simulink model "powerwindow_tl"  (R2021a)
settings: Solver=ode3  StartTime=0.0  StopTime=inf  FixedStep=0.01  RelTol=1e-3  EnableMultiTasking=on
PreLoadFcn:
  | if exist('tl_preloadfcn','file'), tl_preloadfcn(gcs,'5.2.0.25'); end
PostLoadFcn:
  | , if any(exist('dsrtsu_mdlpostloadfcn', 'file') == [2, 3, 6]), try dsrtsu_mdlpostloadfcn('Execute', bdroot); catch fprintf('Error in PostLoadFcn (dsrtsu_mdlpostloadfcn) for model "%s":\n %s\n', bdroot, lasterr); end, end,
  | if exist('tl_postloadfcn','file'), tl_postloadfcn(gcs,'5.2.0.25'); end
InitFcn:
  | , if any(exist('rtifpga_mdlclblib', 'file') ~= 0), rtifpga_mdlclblib('Init', bdroot); end,
  | if exist('tlds_init','file'), tlds_init(gcs); end
StartFcn:
  | if exist('tlds_start','file'), tlds_start(gcs); end
StopFcn:
  | if exist('tlds_stop','file'), tlds_stop(gcs); end
model workspace (MAT data in the model file):
  obs_1 = 1
  obs_10 = 1
  obs_11 = 1
  obs_12 = 1
  obs_13 = 1
  obs_14 = 1
  obs_15 = 1
  obs_16 = 1
  obs_17 = 1
  obs_18 = 1
  obs_19 = 1
  obs_2 = 1
  obs_20 = 1
  obs_21 = 1
  obs_22 = 1
  obs_23 = 1
  obs_24 = 1
  obs_25 = 1
  obs_26 = 1
  obs_27 = 1
  obs_28 = 1
  obs_29 = 1
  obs_3 = 1
  obs_30 = 1
  obs_31 = 1
  obs_32 = 1
  obs_4 = 1
  obs_5 = 1
  obs_6 = 1
  obs_7 = 1
  obs_8 = 1
  obs_9 = 1
values from neighbouring files (symbols this model uses):
  auto_down_time = 100    [powerwindow_tl_init.m]    (also in test_init.m = copy(auto_up_time))
  auto_up_time = 100    [powerwindow_tl_init.m]    (also in test_init.m = Simulink.Parameter)
  emergency_down_time = 100    [powerwindow_tl_init.m]    (also in test_init.m = copy(auto_up_time))
  position_endstop_top = 0.4    [powerwindow_tl_init.m]    (also in test_init.m = Simulink.Parameter)
undefined symbols (not defined in the file or in its folder): DiscIntNeverNeededParam
libraries: tllib x3, powerwindow_blocklib x2
PreSaveFcn:
  | if exist('tl_presavefcn','file'), tl_presavefcn(gcs); end
CloseFcn:
  | if exist('tl_closefcn','file'), tl_closefcn(gcs); end
settings Model: DSRTSU_INTERNAL_RTI_VER=590  DSRTSU_INTERNAL_RTI_TYPE=rti1006  DSRTSU_INTERNAL_RTIFPGA=170  RTICANMMDATA=struct('GeneralSetupData',struct('modelroot','C:\PowerWindowDemo_TL52_22.0J','generalsettings',struct('filesettings',struct('destfolder',struct('Name','RTICANMM_FILES','Check',1),'buildfolder',struct('Name','.','Check',1),'AbsDestfolder',struct('Name','C:\PowerWindowDemo_TL52_22.0J\RTICANMM_FILES'),'AbsBuildfolder',struct('Name','C:\PowerWindowDemo_TL52_22.0J'))),'options',struct('addpaths',1,'rmpaths',1,'addtrcexclusion',true,'cannavigator',struct('checkmonitoring',0),'show_usrtrc',0,'use_usrtrc',0),'advanced',struct('options',ones(1,100)),'MPSetup',{{}},'RTI',struct('Type','ERT','Ver','','Date',''),'modelname','powerwindow_tl','block','powerwindow_tl'))  TL_MAIN_DATA={'date',738790.66649789352}  DS_PROJECTFILE=sample.dd  TLVersion=5.2.0.25  DSRTSU_INTERNAL_RTISTBM_VER=1.4.3  Creator=hholberg  LastModifiedBy=BTCJ_support
settings SolverCC: AlgebraicLoopSolver=TrustRegion
settings DataIOCC: LimitDataPoints=on  SaveFormat=StructureWithTime  ReturnWorkspaceOutputs=off
settings OptimizationCC: BlockReduction=off  OptimizeBlockIOStorage=off  BufferReuse=off  GlobalBufferReuse=off  ExpressionFolding=off  EnableMemcpy=off  ExpressionDepthLimit=2147483647  LocalBlockOutputs=off  ZeroExternalMemoryAtStartup=off  ZeroInternalMemoryAtStartup=off  InitFltsAndDblsToZero=on  LifeSpan=Inf  OptimizeDataStoreBuffers=off  BusAssignmentInplaceUpdate=off  EfficientTunableParamExpr=on
settings DebuggingCC: UnderspecifiedInitializationDetection=Classic  MergeDetectMultiDrivingBlocksExec=none  SolverPrmCheckMsg=warning  FcnCallInpInsideContextMsg=warning  BusObjectLabelMismatch=error  StateNameClashWarn=warning  StrictBusMsg=ErrorOnBusTreatedAsVector  NonBusSignalsTreatedAsBus=error  SFUnexpectedBacktrackingDiag=warning  SFNoUnconditionalDefaultTransitionDiag=warning  SFExecutionAtInitializationDiag=none  SFMachineParentedDataDiag=warning  ArithmeticOperatorsInVariantConditions=warning
settings HardwareCC: ProdBitPerPointer=32  ProdBitPerSizeT=32  ProdBitPerPtrDiffT=32  ProdLargestAtomicInteger=Integer  ProdEndianess=Unspecified  ProdWordSize=32  ProdHWDeviceType=32-bit Generic  TargetIntDivRoundTo=Zero  TargetEndianess=LittleEndian  TargetHWDeviceType=Custom Processor->Custom
settings ModelReferenceCC: PropagateSignalLabelsOutOfModel=off
settings SFSimCC: SimUseLocalCustomCode=off  MATLABDynamicMemAlloc=off  CustomCodeUndefinedFunction=UseInterfaceOnly
settings RTWCC: SystemTargetFile=ert.tlc  GenCodeOnly=on  TemplateMakefile=ert_default_tmf  RTWUseLocalCustomCode=off
settings CodeAppCC: IgnoreCustomStorageClasses=off  StateflowObjectComments=on  InternalIdentifier=Classic
settings ERTTargetCC: MultiwordLength=2048  ERTCustomFileTemplate=example_file_process.tlc  ConvertIfToSwitch=off  SuppressUnreachableDefaultCases=off
settings ConfigComp: CovMetricSettings=dw  CovSaveCumulativeToWorkspaceVar=on  CovSaveSingleToWorkspaceVar=on  CovExternalEMLEnable=off

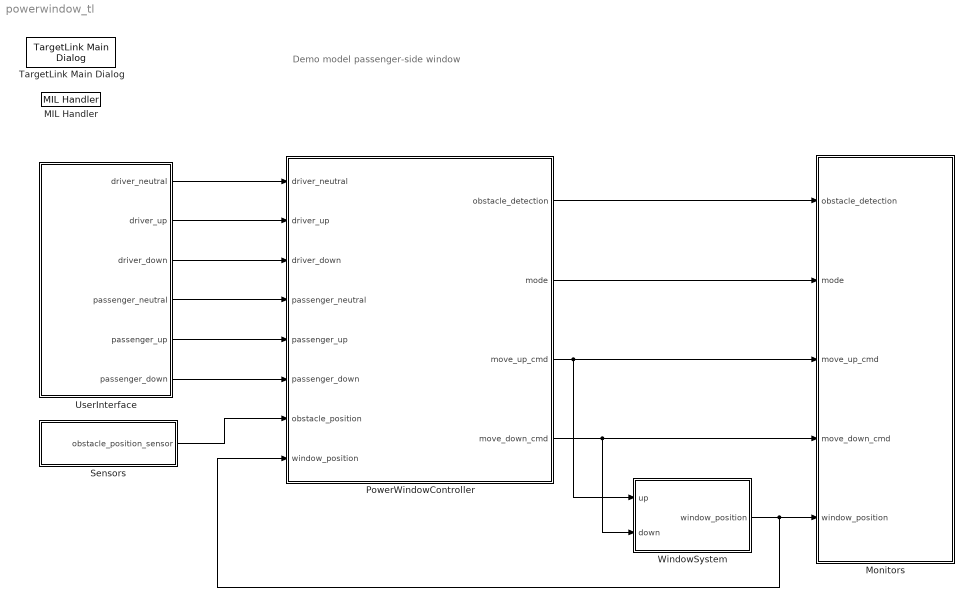
== system powerwindow_tl ==
  note: Demo model passenger-side window
  MIL Handler : tllib/MIL Handler  data={'date',730486}
      settings: SourceProductName=dSPACE TargetLink common blockset
  Monitors : Subsystem
  PowerWindowController : Subsystem  Tag=TargetLink Simulation Frame  mask(TL_SimFrame){}
      settings: CopyFcn=if exist('tl_copyfcn','file'), tl_copyfcn(gcbh); end  NameChangeFcn=if exist('tl_framenamechangefcn','file'), tl_framenamechangefcn(gcbh); end
      settings: OpenFcn=|
      | if exist('open_tlsubsystem','file')
      |    open_tlsubsystem(gcbh);
      | else
      |    tlsubsystem = ...
      |       find_system(gcb, ...
      |       'LookUnderMasks','on', ...
      |       'FollowLinks','on', ...
      |       'Tag','MIL Subsystem');
      |    open_system(tlsubsystem);
      | end
      mask Display: disp('TargetLink\nModel-\nin-the-loop\nmode')
  Sensors : Subsystem
  TargetLink Main Dialog : tllib/TargetLink Main Dialog  data=[]
      settings: SourceProductName=dSPACE TargetLink common blockset
  UserInterface : Subsystem
  WindowSystem : Subsystem
  wires:
  PowerWindowController/3(move_up_cmd) -> WindowSystem/1(up), Monitors/3(move_up_cmd)
  PowerWindowController/4(move_down_cmd) -> Monitors/4(move_down_cmd), WindowSystem/2(down)
  WindowSystem/1(window_position) -> PowerWindowController/8(window_position), Monitors/5(window_position)
  UserInterface/1(driver_neutral) -> PowerWindowController/1(driver_neutral)
  UserInterface/2(driver_up) -> PowerWindowController/2(driver_up)
  UserInterface/3(driver_down) -> PowerWindowController/3(driver_down)
  UserInterface/4(passenger_neutral) -> PowerWindowController/4(passenger_neutral)
  UserInterface/5(passenger_up) -> PowerWindowController/5(passenger_up)
  UserInterface/6(passenger_down) -> PowerWindowController/6(passenger_down)
  Sensors/1(obstacle_position_sensor) -> PowerWindowController/7(obstacle_position)
  PowerWindowController/1(obstacle_detection) -> Monitors/1(obstacle_detection)
  PowerWindowController/2(mode) -> Monitors/2(mode)

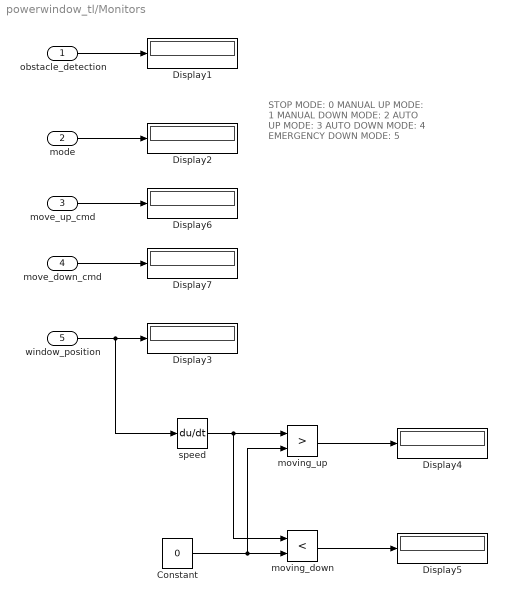
== system powerwindow_tl/Monitors ==
  note: STOP MODE: 0
      | MANUAL UP MODE: 1
      | MANUAL DOWN MODE: 2
      | AUTO UP MODE: 3
      | AUTO DOWN MODE: 4
      | EMERGENCY DOWN MODE: 5
  obstacle_detection : Inport
  mode : Inport  Port=2
  move_up_cmd : Inport  Port=3
  move_down_cmd : Inport  Port=4
  window_position : Inport  Port=5
  Constant : Constant  Value=0
  Display{1..7} (7 alike) : Display
  moving_down : RelationalOperator  Operator=<  OutDataTypeStr=boolean  RndMeth=Nearest
  moving_up : RelationalOperator  Operator=>  OutDataTypeStr=boolean  RndMeth=Nearest
  speed : Derivative
  wires:
  obstacle_detection/1 -> Display1/1
  mode/1 -> Display2/1
  window_position/1 -> speed/1, Display3/1
  speed/1 -> moving_down/1, moving_up/1
  Constant/1 -> moving_down/2, moving_up/2
  moving_down/1 -> Display5/1
  moving_up/1 -> Display4/1
  move_up_cmd/1 -> Display6/1
  move_down_cmd/1 -> Display7/1

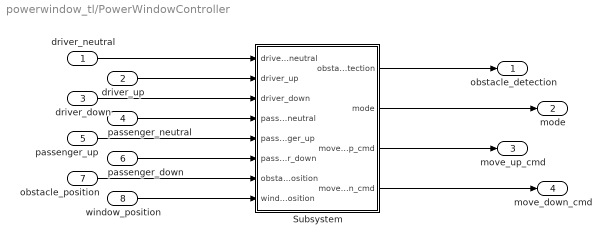
== system powerwindow_tl/PowerWindowController ==
  driver_neutral : Inport
  driver_up : Inport  Port=2
  driver_down : Inport  Port=3
  passenger_neutral : Inport  Port=4
  passenger_up : Inport  Port=5
  passenger_down : Inport  Port=6
  obstacle_position : Inport  Port=7
  window_position : Inport  Port=8
  Subsystem : Subsystem  Tag=struct('sfcnName','PowerWindowController_sf','subFunction','','srcSubsystem','')  mask(TL_Enable){}
      settings: OpenFcn=warndlg(get_param(gcb,'MaskHelp'),'Serious Warning');
      mask Help: This subsystem keeps the TargetLink subsystem (subsystem with TargetLink blocks for production code generation), and is needed for the TargetLink simulation frame to work properly. DO NOT DELETE OR MODIFY IT!
  obstacle_detection : Outport
  mode : Outport  Port=2  OutDataTypeStr=uint8
  move_up_cmd : Outport  Port=3
  move_down_cmd : Outport  Port=4
  wires:
  driver_neutral/1 -> Subsystem/1(driver_neutral)
  driver_up/1 -> Subsystem/2(driver_up)
  driver_down/1 -> Subsystem/3(driver_down)
  passenger_neutral/1 -> Subsystem/4(passenger_neutral)
  passenger_up/1 -> Subsystem/5(passenger_up)
  passenger_down/1 -> Subsystem/6(passenger_down)
  obstacle_position/1 -> Subsystem/7(obstacle_position)
  window_position/1 -> Subsystem/8(window_position)
  Subsystem/1(obstacle_detection) -> obstacle_detection/1
  Subsystem/2(mode) -> mode/1
  Subsystem/3(move_up_cmd) -> move_up_cmd/1
  Subsystem/4(move_down_cmd) -> move_down_cmd/1

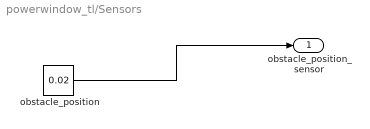
== system powerwindow_tl/Sensors ==
  obstacle_position : Constant  Value=0.02  OutDataTypeStr=double
  obstacle_position_sensor : Outport
  wires:
  obstacle_position/1 -> obstacle_position_sensor/1

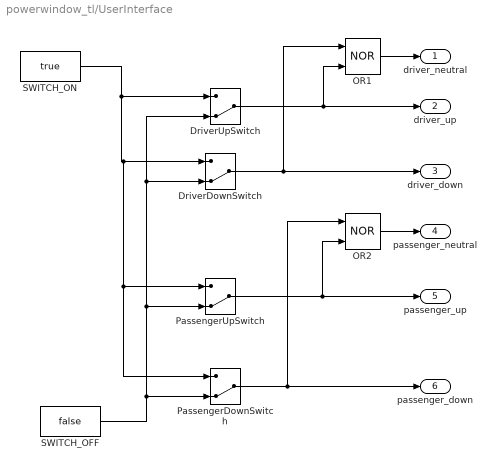
== system powerwindow_tl/UserInterface ==
  DriverDownSwitch : ManualSwitch  CurrentSetting=0
  DriverUpSwitch : ManualSwitch  CurrentSetting=0
  OR1 : Logic  Operator=NOR  AllPortsSameDT=off  OutDataTypeStr=boolean
  OR2 : Logic  Operator=NOR  AllPortsSameDT=off  OutDataTypeStr=boolean
  PassengerDownSwitch : ManualSwitch  CurrentSetting=0
  PassengerUpSwitch : ManualSwitch  CurrentSetting=0
  SWITCH_OFF : Constant  Value=false  OutDataTypeStr=boolean
  SWITCH_ON : Constant  Value=true  OutDataTypeStr=boolean
  driver_neutral : Outport
  driver_up : Outport  Port=2
  driver_down : Outport  Port=3
  passenger_neutral : Outport  Port=4
  passenger_up : Outport  Port=5
  passenger_down : Outport  Port=6
  wires:
  SWITCH_ON/1 -> PassengerDownSwitch/1, PassengerUpSwitch/1, DriverDownSwitch/1, DriverUpSwitch/1
  SWITCH_OFF/1 -> DriverUpSwitch/2, DriverDownSwitch/2, PassengerUpSwitch/2, PassengerDownSwitch/2
  DriverUpSwitch/1 -> OR1/2, driver_up/1
  DriverDownSwitch/1 -> OR1/1, driver_down/1
  OR1/1 -> driver_neutral/1
  PassengerUpSwitch/1 -> OR2/2, passenger_up/1
  PassengerDownSwitch/1 -> OR2/1, passenger_down/1
  OR2/1 -> passenger_neutral/1

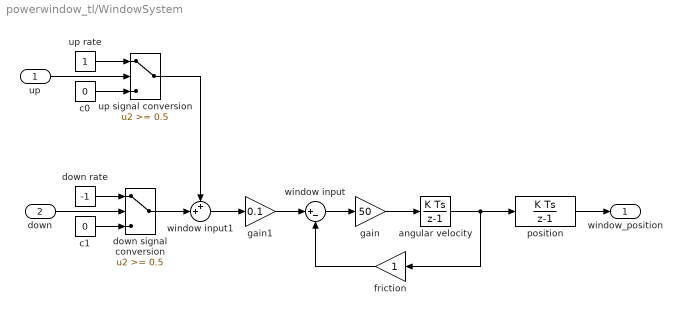
== system powerwindow_tl/WindowSystem ==
  up : Inport
  down : Inport  Port=2
  angular velocity : DiscreteIntegrator  SampleTime=0.01  ICPrevOutput=DiscIntNeverNeededParam  ICPrevScaledInput=DiscIntNeverNeededParam  mask(DiscretizedDiscreteIntegrator){}
      mask init:
      | %zoh
  c0 : Constant  Value=0
  c1 : Constant  Value=0
  down rate : Constant  Value=-1
  down signal conversion : Switch  Threshold=0.5  InputSameDT=on
  friction : Gain  SaturateOnIntegerOverflow=on  OutDataTypeStr=Inherit: Same as input  ParamDataTypeStr=Inherit: Same as input
  gain : Gain  Gain=50  SaturateOnIntegerOverflow=on  OutDataTypeStr=Inherit: Same as input  ParamDataTypeStr=Inherit: Same as input
  gain1 : Gain  Gain=0.1  SaturateOnIntegerOverflow=on  OutDataTypeStr=Inherit: Same as input  ParamDataTypeStr=Inherit: Same as input
  position : DiscreteIntegrator  SampleTime=0.01  LimitOutput=on  UpperSaturationLimit=position_endstop_top  LowerSaturationLimit=0  ICPrevOutput=DiscIntNeverNeededParam  ICPrevScaledInput=DiscIntNeverNeededParam  mask(DiscretizedDiscreteIntegrator){}
      mask init:
      | %zoh
  up rate : Constant
  up signal conversion : Switch  Threshold=0.5  InputSameDT=on
  window input : Sum  Inputs=|+-  InputSameDT=on  SaturateOnIntegerOverflow=on  OutDataTypeStr=Inherit: Same as first input
  window input1 : Sum  Inputs=++|  InputSameDT=on  SaturateOnIntegerOverflow=on  OutDataTypeStr=Inherit: Same as first input
  window_position : Outport
  wires:
  up signal conversion/1 -> window input1/1
  down signal conversion/1 -> window input1/2
  window input1/1 -> gain1/1
  gain1/1 -> window input/1
  down/1 -> down signal conversion/2
  position/1 -> window_position/1
  up/1 -> up signal conversion/2
  up rate/1 -> up signal conversion/1
  c0/1 -> up signal conversion/3
  down rate/1 -> down signal conversion/1
  c1/1 -> down signal conversion/3
  window input/1 -> gain/1
  gain/1 -> angular velocity/1
  angular velocity/1 -> friction/1, position/1
  friction/1 -> window input/2

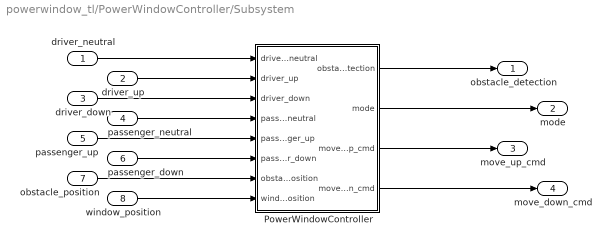
== system powerwindow_tl/PowerWindowController/Subsystem ==
  driver_neutral : Inport
  driver_up : Inport  Port=2
  driver_down : Inport  Port=3
  passenger_neutral : Inport  Port=4
  passenger_up : Inport  Port=5
  passenger_down : Inport  Port=6
  obstacle_position : Inport  Port=7
  window_position : Inport  Port=8
  PowerWindowController : Subsystem  Tag=MIL Subsystem  Description=a  LoadFcn=|  TreatAsAtomicUnit=on
      | if exist('TargetLink.SimFrameHandler.TLSubsystem','class')
      |     TargetLink.SimFrameHandler.TLSubsystem.CreateWatchDog(gcbh);
      | end
      settings: CopyFcn=if exist('tl_copyfcn','file'), tl_copyfcn(gcbh); end  NameChangeFcn=if exist('tl_namechangefcn','file'), tl_namechangefcn(gcbh); end  DestroyFcn=if exist('update_tl_main_dlg','file'), update_tl_main_dlg('TL_subs_display'); end
      mask Display: disp('TargetLink Subsystem')
  obstacle_detection : Outport
  mode : Outport  Port=2
  move_up_cmd : Outport  Port=3
  move_down_cmd : Outport  Port=4
  wires:
  driver_neutral/1 -> PowerWindowController/1(driver_neutral)
  driver_up/1 -> PowerWindowController/2(driver_up)
  driver_down/1 -> PowerWindowController/3(driver_down)
  passenger_neutral/1 -> PowerWindowController/4(passenger_neutral)
  passenger_up/1 -> PowerWindowController/5(passenger_up)
  passenger_down/1 -> PowerWindowController/6(passenger_down)
  obstacle_position/1 -> PowerWindowController/7(obstacle_position)
  window_position/1 -> PowerWindowController/8(window_position)
  PowerWindowController/1(obstacle_detection) -> obstacle_detection/1
  PowerWindowController/2(mode) -> mode/1
  PowerWindowController/3(move_up_cmd) -> move_up_cmd/1
  PowerWindowController/4(move_down_cmd) -> move_down_cmd/1

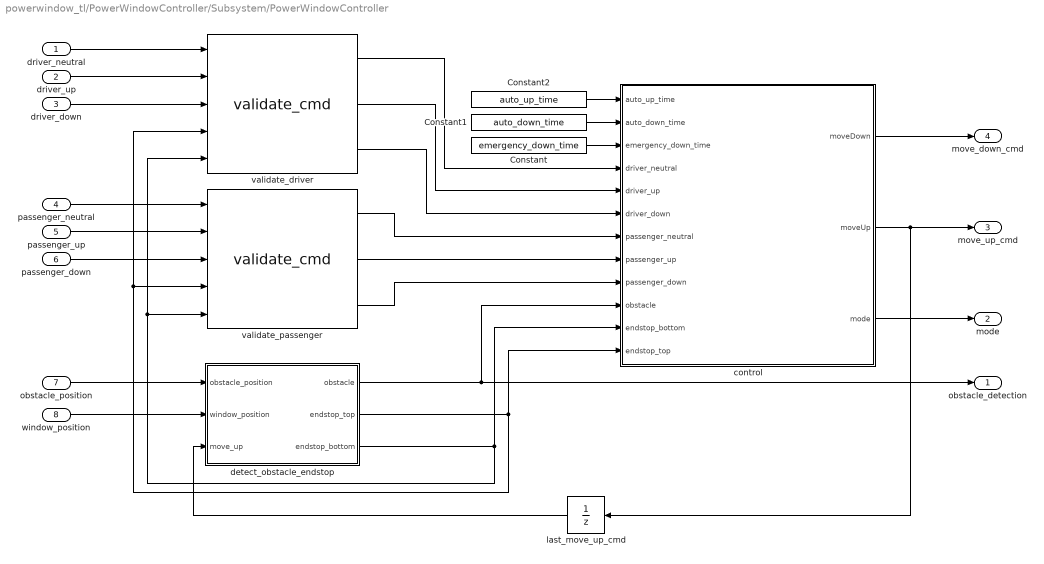
== system powerwindow_tl/PowerWindowController/Subsystem/PowerWindowController ==
  driver_neutral : Inport  PortDimensions=1  mask(TL_Inport){data={'output',{'type','Bool'},'date',738295.41950233793}}
      settings: CopyFcn=if exist('copy_tlblock','file')==2,copy_tlblock(gcbh);end  DeleteFcn=if exist('delete_tlblock','file')==2,delete_tlblock(gcbh);end  NameChangeFcn=if exist('rename_tlblock','file')==2,rename_tlblock(gcbh);end  OpenFcn=if exist('tl_open_blockdlg','file')==2,tl_open_blockdlg(gcbh);else,open_system(gcbh,'parameter');end
      mask Help: eval(['if exist(''tl_online_help'',''file'') == 2, tl_online_help(''Topic'',''TL_Inport''),else, web([''jar:file:///'',matlabroot,''/help/toolbox/simulink/help.jar!/slref/' lower(get_param(gcbh,'Blocktype')) '.html''], ''-helpbrowser''),end'])
      mask Display:
      | [x,y] = tlDrawBrandOnBlockIcon(gcbh);
      | plot(x,y);
  driver_up : Inport  Port=2  PortDimensions=1  mask(TL_Inport){data={'output',{'type','Bool'},'date',738295.4195026157}}
      settings: CopyFcn=if exist('copy_tlblock','file')==2,copy_tlblock(gcbh);end  DeleteFcn=if exist('delete_tlblock','file')==2,delete_tlblock(gcbh);end  NameChangeFcn=if exist('rename_tlblock','file')==2,rename_tlblock(gcbh);end  OpenFcn=if exist('tl_open_blockdlg','file')==2,tl_open_blockdlg(gcbh);else,open_system(gcbh,'parameter');end
      mask Help: eval(['if exist(''tl_online_help'',''file'') == 2, tl_online_help(''Topic'',''TL_Inport''),else, web([''jar:file:///'',matlabroot,''/help/toolbox/simulink/help.jar!/slref/' lower(get_param(gcbh,'Blocktype')) '.html''], ''-helpbrowser''),end'])
      mask Display:
      | [x,y] = tlDrawBrandOnBlockIcon(gcbh);
      | plot(x,y);
  driver_down : Inport  Port=3  PortDimensions=1  mask(TL_Inport){data={'output',{'type','Bool'},'date',738295.41950276622}}
      settings: CopyFcn=if exist('copy_tlblock','file')==2,copy_tlblock(gcbh);end  DeleteFcn=if exist('delete_tlblock','file')==2,delete_tlblock(gcbh);end  NameChangeFcn=if exist('rename_tlblock','file')==2,rename_tlblock(gcbh);end  OpenFcn=if exist('tl_open_blockdlg','file')==2,tl_open_blockdlg(gcbh);else,open_system(gcbh,'parameter');end
      mask Help: eval(['if exist(''tl_online_help'',''file'') == 2, tl_online_help(''Topic'',''TL_Inport''),else, web([''jar:file:///'',matlabroot,''/help/toolbox/simulink/help.jar!/slref/' lower(get_param(gcbh,'Blocktype')) '.html''], ''-helpbrowser''),end'])
      mask Display:
      | [x,y] = tlDrawBrandOnBlockIcon(gcbh);
      | plot(x,y);
  passenger_neutral : Inport  Port=4  PortDimensions=1  mask(TL_Inport){data={'output',{'type','Bool'},'date',738295.41950287041}}
      settings: CopyFcn=if exist('copy_tlblock','file')==2,copy_tlblock(gcbh);end  DeleteFcn=if exist('delete_tlblock','file')==2,delete_tlblock(gcbh);end  NameChangeFcn=if exist('rename_tlblock','file')==2,rename_tlblock(gcbh);end  OpenFcn=if exist('tl_open_blockdlg','file')==2,tl_open_blockdlg(gcbh);else,open_system(gcbh,'parameter');end
      mask Help: eval(['if exist(''tl_online_help'',''file'') == 2, tl_online_help(''Topic'',''TL_Inport''),else, web([''jar:file:///'',matlabroot,''/help/toolbox/simulink/help.jar!/slref/' lower(get_param(gcbh,'Blocktype')) '.html''], ''-helpbrowser''),end'])
      mask Display:
      | [x,y] = tlDrawBrandOnBlockIcon(gcbh);
      | plot(x,y);
  passenger_up : Inport  Port=5  PortDimensions=1  mask(TL_Inport){data={'output',{'type','Bool'},'date',738295.41950299765}}
      settings: CopyFcn=if exist('copy_tlblock','file')==2,copy_tlblock(gcbh);end  DeleteFcn=if exist('delete_tlblock','file')==2,delete_tlblock(gcbh);end  NameChangeFcn=if exist('rename_tlblock','file')==2,rename_tlblock(gcbh);end  OpenFcn=if exist('tl_open_blockdlg','file')==2,tl_open_blockdlg(gcbh);else,open_system(gcbh,'parameter');end
      mask Help: eval(['if exist(''tl_online_help'',''file'') == 2, tl_online_help(''Topic'',''TL_Inport''),else, web([''jar:file:///'',matlabroot,''/help/toolbox/simulink/help.jar!/slref/' lower(get_param(gcbh,'Blocktype')) '.html''], ''-helpbrowser''),end'])
      mask Display:
      | [x,y] = tlDrawBrandOnBlockIcon(gcbh);
      | plot(x,y);
  passenger_down : Inport  Port=6  PortDimensions=1  mask(TL_Inport){data={'output',{'type','Bool'},'date',738295.41950309032}}
      settings: CopyFcn=if exist('copy_tlblock','file')==2,copy_tlblock(gcbh);end  DeleteFcn=if exist('delete_tlblock','file')==2,delete_tlblock(gcbh);end  NameChangeFcn=if exist('rename_tlblock','file')==2,rename_tlblock(gcbh);end  OpenFcn=if exist('tl_open_blockdlg','file')==2,tl_open_blockdlg(gcbh);else,open_system(gcbh,'parameter');end
      mask Help: eval(['if exist(''tl_online_help'',''file'') == 2, tl_online_help(''Topic'',''TL_Inport''),else, web([''jar:file:///'',matlabroot,''/help/toolbox/simulink/help.jar!/slref/' lower(get_param(gcbh,'Blocktype')) '.html''], ''-helpbrowser''),end'])
      mask Display:
      | [x,y] = tlDrawBrandOnBlockIcon(gcbh);
      | plot(x,y);
  obstacle_position : Inport  Port=7  PortDimensions=1  mask(TL_Inport){data={'output',{'max',1,'min',0,'type','UInt16','scaling','SC_Pos'},'date',738295.41950320604}}
      settings: CopyFcn=if exist('copy_tlblock','file')==2,copy_tlblock(gcbh);end  DeleteFcn=if exist('delete_tlblock','file')==2,delete_tlblock(gcbh);end  NameChangeFcn=if exist('rename_tlblock','file')==2,rename_tlblock(gcbh);end  OpenFcn=if exist('tl_open_blockdlg','file')==2,tl_open_blockdlg(gcbh);else,open_system(gcbh,'parameter');end
      mask Help: eval(['if exist(''tl_online_help'',''file'') == 2, tl_online_help(''Topic'',''TL_Inport''),else, web([''jar:file:///'',matlabroot,''/help/toolbox/simulink/help.jar!/slref/' lower(get_param(gcbh,'Blocktype')) '.html''], ''-helpbrowser''),end'])
      mask Display:
      | [x,y] = tlDrawBrandOnBlockIcon(gcbh);
      | plot(x,y);
  window_position : Inport  Port=8  PortDimensions=1  mask(TL_Inport){data={'output',{'max',1,'min',0,'type','UInt16','scaling','SC_Pos'},'date',738295.41950332175}}
      settings: CopyFcn=if exist('copy_tlblock','file')==2,copy_tlblock(gcbh);end  DeleteFcn=if exist('delete_tlblock','file')==2,delete_tlblock(gcbh);end  NameChangeFcn=if exist('rename_tlblock','file')==2,rename_tlblock(gcbh);end  OpenFcn=if exist('tl_open_blockdlg','file')==2,tl_open_blockdlg(gcbh);else,open_system(gcbh,'parameter');end
      mask Help: eval(['if exist(''tl_online_help'',''file'') == 2, tl_online_help(''Topic'',''TL_Inport''),else, web([''jar:file:///'',matlabroot,''/help/toolbox/simulink/help.jar!/slref/' lower(get_param(gcbh,'Blocktype')) '.html''], ''-helpbrowser''),end'])
      mask Display:
      | [x,y] = tlDrawBrandOnBlockIcon(gcbh);
      | plot(x,y);
  Constant : Constant  Value=emergency_down_time  mask(TL_Constant){data={'output',{'variable','emergency_down_time'},'date',736551.41282901622}}
      settings: CopyFcn=if exist('copy_tlblock','file')==2,copy_tlblock(gcbh);end  DeleteFcn=if exist('delete_tlblock','file')==2,delete_tlblock(gcbh);end  NameChangeFcn=if exist('rename_tlblock','file')==2,rename_tlblock(gcbh);end  OpenFcn=if exist('tl_open_blockdlg','file')==2,tl_open_blockdlg(gcbh);else,open_system(gcbh,'parameter');end
      mask Help: eval(['if exist(''tl_online_help'',''file'') == 2, tl_online_help(''Topic'',''TL_Constant''),else, web([''jar:file:///'',matlabroot,''/help/toolbox/simulink/help.jar!/slref/' lower(get_param(gcbh,'Blocktype')) '.html''], ''-helpbrowser''),end'])
      mask Display:
      | [x,y] = tlDrawBrandOnBlockIcon(gcbh);
      | plot(x,y);
  Constant1 : Constant  Value=auto_down_time  mask(TL_Constant){data={'output',{'variable','auto_down_time'},'date',736551.41273832181}}
      settings: CopyFcn=if exist('copy_tlblock','file')==2,copy_tlblock(gcbh);end  DeleteFcn=if exist('delete_tlblock','file')==2,delete_tlblock(gcbh);end  NameChangeFcn=if exist('rename_tlblock','file')==2,rename_tlblock(gcbh);end  OpenFcn=if exist('tl_open_blockdlg','file')==2,tl_open_blockdlg(gcbh);else,open_system(gcbh,'parameter');end
      mask Help: eval(['if exist(''tl_online_help'',''file'') == 2, tl_online_help(''Topic'',''TL_Constant''),else, web([''jar:file:///'',matlabroot,''/help/toolbox/simulink/help.jar!/slref/' lower(get_param(gcbh,'Blocktype')) '.html''], ''-helpbrowser''),end'])
      mask Display:
      | [x,y] = tlDrawBrandOnBlockIcon(gcbh);
      | plot(x,y);
  Constant2 : Constant  Value=auto_up_time  mask(TL_Constant){data={'output',{'variable','auto_up_time'},'date',736551.41214959486}}
      settings: CopyFcn=if exist('copy_tlblock','file')==2,copy_tlblock(gcbh);end  DeleteFcn=if exist('delete_tlblock','file')==2,delete_tlblock(gcbh);end  NameChangeFcn=if exist('rename_tlblock','file')==2,rename_tlblock(gcbh);end  OpenFcn=if exist('tl_open_blockdlg','file')==2,tl_open_blockdlg(gcbh);else,open_system(gcbh,'parameter');end
      mask Help: eval(['if exist(''tl_online_help'',''file'') == 2, tl_online_help(''Topic'',''TL_Constant''),else, web([''jar:file:///'',matlabroot,''/help/toolbox/simulink/help.jar!/slref/' lower(get_param(gcbh,'Blocktype')) '.html''], ''-helpbrowser''),end'])
      mask Display:
      | [x,y] = tlDrawBrandOnBlockIcon(gcbh);
      | plot(x,y);
  control : Stateflow chart  RequirementInfo={} %GIDa_8bba6e11_babd_460a_9a10_505c5c55b95f  TreatAsAtomicUnit=on
  detect_obstacle_endstop : Subsystem  TreatAsAtomicUnit=on
  last_move_up_cmd : UnitDelay  SampleTime=-1  HasFrameUpgradeWarning=on  mask(TL_UnitDelay){data={'output',{'variable','move_up_cmd'},'state',{'type','Bool'},'date',738791.46739337966}}
      settings: CopyFcn=if exist('copy_tlblock','file')==2,copy_tlblock(gcbh);end  DeleteFcn=if exist('delete_tlblock','file')==2,delete_tlblock(gcbh);end  NameChangeFcn=if exist('rename_tlblock','file')==2,rename_tlblock(gcbh);end  OpenFcn=if exist('tl_open_blockdlg','file')==2,tl_open_blockdlg(gcbh);else,open_system(gcbh,'parameter');end
      mask Help: eval(['if exist(''tl_online_help'',''file'') == 2, tl_online_help(''Topic'',''TL_UnitDelay''),else, web([''jar:file:///'',matlabroot,''/help/toolbox/simulink/help.jar!/slref/' lower(get_param(gcbh,'Blocktype')) '.html''], ''-helpbrowser''),end'])
      mask Display:
      | [x,y] = tlDrawBrandOnBlockIcon(gcbh);
      | plot(x,y);
  validate_driver : powerwindow_blocklib/validate_cmd  SystemSampleTime=-1  VariantActivationTime=update diagram  Latency=0  AutoFrameSizeCalculation=off
  validate_passenger : powerwindow_blocklib/validate_cmd  SystemSampleTime=-1  VariantActivationTime=update diagram  Latency=0  AutoFrameSizeCalculation=off
  obstacle_detection : Outport  PortDimensions=1  mask(TL_Outport){data={'output',{'type','Bool'},'date',738295.41950025468}}
      settings: CopyFcn=if exist('copy_tlblock','file')==2,copy_tlblock(gcbh);end  DeleteFcn=if exist('delete_tlblock','file')==2,delete_tlblock(gcbh);end  NameChangeFcn=if exist('rename_tlblock','file')==2,rename_tlblock(gcbh);end  OpenFcn=if exist('tl_open_blockdlg','file')==2,tl_open_blockdlg(gcbh);else,open_system(gcbh,'parameter');end
      mask Help: eval(['if exist(''tl_online_help'',''file'') == 2, tl_online_help(''Topic'',''TL_Outport''),else, web([''jar:file:///'',matlabroot,''/help/toolbox/simulink/help.jar!/slref/' lower(get_param(gcbh,'Blocktype')) '.html''], ''-helpbrowser''),end'])
      mask Display:
      | [x,y] = tlDrawBrandOnBlockIcon(gcbh);
      | plot(x,y);
  mode : Outport  Port=2  OutDataTypeStr=uint8  PortDimensions=1  mask(TL_Outport){data={'output',{'type','UInt8'},'date',738295.41950122686}}
      settings: CopyFcn=if exist('copy_tlblock','file')==2,copy_tlblock(gcbh);end  DeleteFcn=if exist('delete_tlblock','file')==2,delete_tlblock(gcbh);end  NameChangeFcn=if exist('rename_tlblock','file')==2,rename_tlblock(gcbh);end  OpenFcn=if exist('tl_open_blockdlg','file')==2,tl_open_blockdlg(gcbh);else,open_system(gcbh,'parameter');end
      mask Help: eval(['if exist(''tl_online_help'',''file'') == 2, tl_online_help(''Topic'',''TL_Outport''),else, web([''jar:file:///'',matlabroot,''/help/toolbox/simulink/help.jar!/slref/' lower(get_param(gcbh,'Blocktype')) '.html''], ''-helpbrowser''),end'])
      mask Display:
      | [x,y] = tlDrawBrandOnBlockIcon(gcbh);
      | plot(x,y);
  move_up_cmd : Outport  Port=3  PortDimensions=1  mask(TL_Outport){data={'output',{'variable','move_up_cmd'},'date',738295.41950155096}}
      settings: CopyFcn=if exist('copy_tlblock','file')==2,copy_tlblock(gcbh);end  DeleteFcn=if exist('delete_tlblock','file')==2,delete_tlblock(gcbh);end  NameChangeFcn=if exist('rename_tlblock','file')==2,rename_tlblock(gcbh);end  OpenFcn=if exist('tl_open_blockdlg','file')==2,tl_open_blockdlg(gcbh);else,open_system(gcbh,'parameter');end
      mask Help: eval(['if exist(''tl_online_help'',''file'') == 2, tl_online_help(''Topic'',''TL_Outport''),else, web([''jar:file:///'',matlabroot,''/help/toolbox/simulink/help.jar!/slref/' lower(get_param(gcbh,'Blocktype')) '.html''], ''-helpbrowser''),end'])
      mask Display:
      | [x,y] = tlDrawBrandOnBlockIcon(gcbh);
      | plot(x,y);
  move_down_cmd : Outport  Port=4  PortDimensions=1  mask(TL_Outport){data={'output',{'variable','move_down_cmd'},'date',738295.41950209485}}
      settings: CopyFcn=if exist('copy_tlblock','file')==2,copy_tlblock(gcbh);end  DeleteFcn=if exist('delete_tlblock','file')==2,delete_tlblock(gcbh);end  NameChangeFcn=if exist('rename_tlblock','file')==2,rename_tlblock(gcbh);end  OpenFcn=if exist('tl_open_blockdlg','file')==2,tl_open_blockdlg(gcbh);else,open_system(gcbh,'parameter');end
      mask Help: eval(['if exist(''tl_online_help'',''file'') == 2, tl_online_help(''Topic'',''TL_Outport''),else, web([''jar:file:///'',matlabroot,''/help/toolbox/simulink/help.jar!/slref/' lower(get_param(gcbh,'Blocktype')) '.html''], ''-helpbrowser''),end'])
      mask Display:
      | [x,y] = tlDrawBrandOnBlockIcon(gcbh);
      | plot(x,y);
  wires:
  control/3(mode) -> mode/1
  Constant2/1 -> control/1(auto_up_time)
  Constant1/1 -> control/2(auto_down_time)
  Constant/1 -> control/3(emergency_down_time)
  detect_obstacle_endstop/2(endstop_top) -> control/12(endstop_top), validate_passenger/4, validate_driver/4
  detect_obstacle_endstop/3(endstop_bottom) -> control/11(endstop_bottom), validate_passenger/5, validate_driver/5
  validate_driver/3 -> control/6(driver_down)
  validate_passenger/3 -> control/9(passenger_down)
  validate_passenger/2 -> control/8(passenger_up)
  validate_passenger/1 -> control/7(passenger_neutral)
  control/2(moveUp) -> last_move_up_cmd/1, move_up_cmd/1
  validate_driver/2 -> control/5(driver_up)
  validate_driver/1 -> control/4(driver_neutral)
  detect_obstacle_endstop/1(obstacle) -> control/10(obstacle), obstacle_detection/1
  control/1(moveDown) -> move_down_cmd/1
  driver_neutral/1 -> validate_driver/1
  driver_up/1 -> validate_driver/2
  driver_down/1 -> validate_driver/3
  passenger_neutral/1 -> validate_passenger/1
  passenger_up/1 -> validate_passenger/2
  passenger_down/1 -> validate_passenger/3
  last_move_up_cmd/1 -> detect_obstacle_endstop/3(move_up)
  obstacle_position/1 -> detect_obstacle_endstop/1(obstacle_position)
  window_position/1 -> detect_obstacle_endstop/2(window_position)

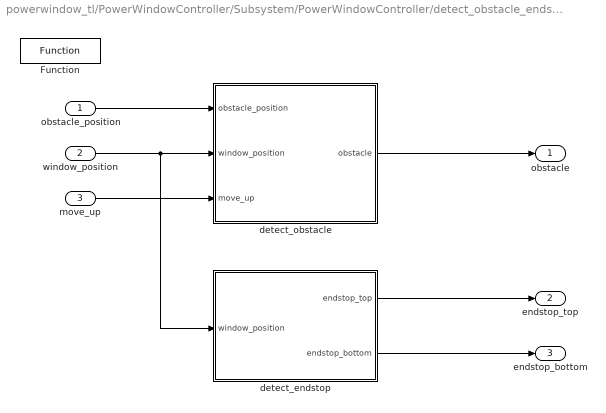
== system powerwindow_tl/PowerWindowController/Subsystem/PowerWindowController/detect_obstacle_endstop ==
  obstacle_position : Inport
  window_position : Inport  Port=2
  move_up : Inport  Port=3
  Function : tllib/Function  data={'date',738295.4195037731}  displayString=FUNCTION
      settings: SourceProductName=dSPACE TargetLink common blockset
  detect_endstop : Subsystem
  detect_obstacle : Subsystem
  obstacle : Outport
  endstop_top : Outport  Port=2
  endstop_bottom : Outport  Port=3
  wires:
  detect_endstop/2(endstop_bottom) -> endstop_bottom/1
  detect_endstop/1(endstop_top) -> endstop_top/1
  move_up/1 -> detect_obstacle/3(move_up)
  window_position/1 -> detect_endstop/1(window_position), detect_obstacle/2(window_position)
  obstacle_position/1 -> detect_obstacle/1(obstacle_position)
  detect_obstacle/1(obstacle) -> obstacle/1

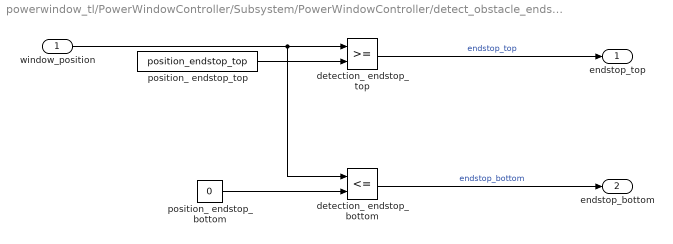
== system powerwindow_tl/PowerWindowController/Subsystem/PowerWindowController/detect_obstacle_endstop/detect_endstop ==
  window_position : Inport
  detection_ endstop_bottom : RelationalOperator  Operator=<=  OutDataTypeStr=boolean  RndMeth=Nearest  InputSameDT=on  mask(TL_RelationalOperator){data={'date',736551.40566996532}}
      settings: CopyFcn=if exist('copy_tlblock','file')==2,copy_tlblock(gcbh);end  DeleteFcn=if exist('delete_tlblock','file')==2,delete_tlblock(gcbh);end  NameChangeFcn=if exist('rename_tlblock','file')==2,rename_tlblock(gcbh);end  OpenFcn=if exist('tl_open_blockdlg','file')==2,tl_open_blockdlg(gcbh);else,open_system(gcbh,'parameter');end
      mask Help: eval(['if exist(''tl_online_help'',''file'') == 2, tl_online_help(''Topic'',''TL_RelationalOperator''),else, web([''jar:file:///'',matlabroot,''/help/toolbox/simulink/help.jar!/slref/' lower(get_param(gcbh,'Blocktype')) '.html''], ''-helpbrowser''),end'])
      mask Display:
      | [x,y] = tlDrawBrandOnBlockIcon(gcbh);
      | plot(x,y);
  detection_ endstop_top : RelationalOperator  OutDataTypeStr=boolean  RndMeth=Nearest  InputSameDT=on  mask(TL_RelationalOperator){data={'date',736551.40567012737}}
      settings: CopyFcn=if exist('copy_tlblock','file')==2,copy_tlblock(gcbh);end  DeleteFcn=if exist('delete_tlblock','file')==2,delete_tlblock(gcbh);end  NameChangeFcn=if exist('rename_tlblock','file')==2,rename_tlblock(gcbh);end  OpenFcn=if exist('tl_open_blockdlg','file')==2,tl_open_blockdlg(gcbh);else,open_system(gcbh,'parameter');end
      mask Help: eval(['if exist(''tl_online_help'',''file'') == 2, tl_online_help(''Topic'',''TL_RelationalOperator''),else, web([''jar:file:///'',matlabroot,''/help/toolbox/simulink/help.jar!/slref/' lower(get_param(gcbh,'Blocktype')) '.html''], ''-helpbrowser''),end'])
      mask Display:
      | [x,y] = tlDrawBrandOnBlockIcon(gcbh);
      | plot(x,y);
  position_ endstop_bottom : Constant  Value=0  mask(TL_Constant){data={'date',736551.40567030094}}
      settings: CopyFcn=if exist('copy_tlblock','file')==2,copy_tlblock(gcbh);end  DeleteFcn=if exist('delete_tlblock','file')==2,delete_tlblock(gcbh);end  NameChangeFcn=if exist('rename_tlblock','file')==2,rename_tlblock(gcbh);end  OpenFcn=if exist('tl_open_blockdlg','file')==2,tl_open_blockdlg(gcbh);else,open_system(gcbh,'parameter');end
      mask Help: eval(['if exist(''tl_online_help'',''file'') == 2, tl_online_help(''Topic'',''TL_Constant''),else, web([''jar:file:///'',matlabroot,''/help/toolbox/simulink/help.jar!/slref/' lower(get_param(gcbh,'Blocktype')) '.html''], ''-helpbrowser''),end'])
      mask Display:
      | [x,y] = tlDrawBrandOnBlockIcon(gcbh);
      | plot(x,y);
  position_ endstop_top : Constant  Value=position_endstop_top  mask(TL_Constant){data={'output',{'variable','position_endstop_top'},'date',736551.4102625231}}
      settings: CopyFcn=if exist('copy_tlblock','file')==2,copy_tlblock(gcbh);end  DeleteFcn=if exist('delete_tlblock','file')==2,delete_tlblock(gcbh);end  NameChangeFcn=if exist('rename_tlblock','file')==2,rename_tlblock(gcbh);end  OpenFcn=if exist('tl_open_blockdlg','file')==2,tl_open_blockdlg(gcbh);else,open_system(gcbh,'parameter');end
      mask Help: eval(['if exist(''tl_online_help'',''file'') == 2, tl_online_help(''Topic'',''TL_Constant''),else, web([''jar:file:///'',matlabroot,''/help/toolbox/simulink/help.jar!/slref/' lower(get_param(gcbh,'Blocktype')) '.html''], ''-helpbrowser''),end'])
      mask Display:
      | [x,y] = tlDrawBrandOnBlockIcon(gcbh);
      | plot(x,y);
  endstop_top : Outport
  endstop_bottom : Outport  Port=2
  wires:
  position_ endstop_top/1 -> detection_ endstop_top/2
  detection_ endstop_bottom/1 -> endstop_bottom/1  "endstop_bottom"
  detection_ endstop_top/1 -> endstop_top/1  "endstop_top"
  window_position/1 -> detection_ endstop_top/1, detection_ endstop_bottom/1
  position_ endstop_bottom/1 -> detection_ endstop_bottom/2

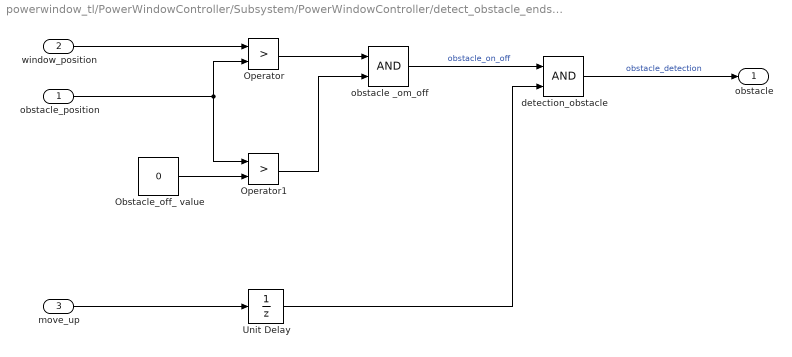
== system powerwindow_tl/PowerWindowController/Subsystem/PowerWindowController/detect_obstacle_endstop/detect_obstacle ==
  obstacle_position : Inport
  window_position : Inport  Port=2
  move_up : Inport  Port=3
  Obstacle_off_ value : Constant  Value=0  mask(TL_Constant){data={'date',736551.40567067126}}
      settings: CopyFcn=if exist('copy_tlblock','file')==2,copy_tlblock(gcbh);end  DeleteFcn=if exist('delete_tlblock','file')==2,delete_tlblock(gcbh);end  NameChangeFcn=if exist('rename_tlblock','file')==2,rename_tlblock(gcbh);end  OpenFcn=if exist('tl_open_blockdlg','file')==2,tl_open_blockdlg(gcbh);else,open_system(gcbh,'parameter');end
      mask Help: eval(['if exist(''tl_online_help'',''file'') == 2, tl_online_help(''Topic'',''TL_Constant''),else, web([''jar:file:///'',matlabroot,''/help/toolbox/simulink/help.jar!/slref/' lower(get_param(gcbh,'Blocktype')) '.html''], ''-helpbrowser''),end'])
      mask Display:
      | [x,y] = tlDrawBrandOnBlockIcon(gcbh);
      | plot(x,y);
  Operator : RelationalOperator  Operator=>  OutDataTypeStr=boolean  RndMeth=Nearest  InputSameDT=on  mask(TL_RelationalOperator){data={'date',736551.40567081014}}
      settings: CopyFcn=if exist('copy_tlblock','file')==2,copy_tlblock(gcbh);end  DeleteFcn=if exist('delete_tlblock','file')==2,delete_tlblock(gcbh);end  NameChangeFcn=if exist('rename_tlblock','file')==2,rename_tlblock(gcbh);end  OpenFcn=if exist('tl_open_blockdlg','file')==2,tl_open_blockdlg(gcbh);else,open_system(gcbh,'parameter');end
      mask Help: eval(['if exist(''tl_online_help'',''file'') == 2, tl_online_help(''Topic'',''TL_RelationalOperator''),else, web([''jar:file:///'',matlabroot,''/help/toolbox/simulink/help.jar!/slref/' lower(get_param(gcbh,'Blocktype')) '.html''], ''-helpbrowser''),end'])
      mask Display:
      | [x,y] = tlDrawBrandOnBlockIcon(gcbh);
      | plot(x,y);
  Operator1 : RelationalOperator  Operator=>  OutDataTypeStr=boolean  RndMeth=Nearest  InputSameDT=on  mask(TL_RelationalOperator){data={'date',736551.40567097219}}
      settings: CopyFcn=if exist('copy_tlblock','file')==2,copy_tlblock(gcbh);end  DeleteFcn=if exist('delete_tlblock','file')==2,delete_tlblock(gcbh);end  NameChangeFcn=if exist('rename_tlblock','file')==2,rename_tlblock(gcbh);end  OpenFcn=if exist('tl_open_blockdlg','file')==2,tl_open_blockdlg(gcbh);else,open_system(gcbh,'parameter');end
      mask Help: eval(['if exist(''tl_online_help'',''file'') == 2, tl_online_help(''Topic'',''TL_RelationalOperator''),else, web([''jar:file:///'',matlabroot,''/help/toolbox/simulink/help.jar!/slref/' lower(get_param(gcbh,'Blocktype')) '.html''], ''-helpbrowser''),end'])
      mask Display:
      | [x,y] = tlDrawBrandOnBlockIcon(gcbh);
      | plot(x,y);
  Unit Delay : UnitDelay  SampleTime=-1  HasFrameUpgradeWarning=on  mask(TL_UnitDelay){data={'output',{'variable','move_up_cmd'},'state',{'type','Bool'},'date',737383.60909223382}}
      settings: CopyFcn=if exist('copy_tlblock','file')==2,copy_tlblock(gcbh);end  DeleteFcn=if exist('delete_tlblock','file')==2,delete_tlblock(gcbh);end  NameChangeFcn=if exist('rename_tlblock','file')==2,rename_tlblock(gcbh);end  OpenFcn=if exist('tl_open_blockdlg','file')==2,tl_open_blockdlg(gcbh);else,open_system(gcbh,'parameter');end
      mask Help: eval(['if exist(''tl_online_help'',''file'') == 2, tl_online_help(''Topic'',''TL_UnitDelay''),else, web([''jar:file:///'',matlabroot,''/help/toolbox/simulink/help.jar!/slref/' lower(get_param(gcbh,'Blocktype')) '.html''], ''-helpbrowser''),end'])
      mask Display:
      | [x,y] = tlDrawBrandOnBlockIcon(gcbh);
      | plot(x,y);
  detection_obstacle : Logic  AllPortsSameDT=off  OutDataTypeStr=boolean  mask(TL_LogicalOperator){data={'date',736551.40567170142}}
      settings: CopyFcn=if exist('copy_tlblock','file')==2,copy_tlblock(gcbh);end  DeleteFcn=if exist('delete_tlblock','file')==2,delete_tlblock(gcbh);end  NameChangeFcn=if exist('rename_tlblock','file')==2,rename_tlblock(gcbh);end  OpenFcn=if exist('tl_open_blockdlg','file')==2,tl_open_blockdlg(gcbh);else,open_system(gcbh,'parameter');end
      mask Help: eval(['if exist(''tl_online_help'',''file'') == 2, tl_online_help(''Topic'',''TL_LogicalOperator''),else, web([''jar:file:///'',matlabroot,''/help/toolbox/simulink/help.jar!/slref/' lower(get_param(gcbh,'Blocktype')) '.html''], ''-helpbrowser''),end'])
      mask Display:
      | [x,y] = tlDrawBrandOnBlockIcon(gcbh);
      | plot(x,y);
  obstacle _om_off : Logic  AllPortsSameDT=off  OutDataTypeStr=boolean  mask(TL_LogicalOperator){data={'date',736551.40567187499}}
      settings: CopyFcn=if exist('copy_tlblock','file')==2,copy_tlblock(gcbh);end  DeleteFcn=if exist('delete_tlblock','file')==2,delete_tlblock(gcbh);end  NameChangeFcn=if exist('rename_tlblock','file')==2,rename_tlblock(gcbh);end  OpenFcn=if exist('tl_open_blockdlg','file')==2,tl_open_blockdlg(gcbh);else,open_system(gcbh,'parameter');end
      mask Help: eval(['if exist(''tl_online_help'',''file'') == 2, tl_online_help(''Topic'',''TL_LogicalOperator''),else, web([''jar:file:///'',matlabroot,''/help/toolbox/simulink/help.jar!/slref/' lower(get_param(gcbh,'Blocktype')) '.html''], ''-helpbrowser''),end'])
      mask Display:
      | [x,y] = tlDrawBrandOnBlockIcon(gcbh);
      | plot(x,y);
  obstacle : Outport
  wires:
  obstacle _om_off/1 -> detection_obstacle/1  "obstacle_on_off"
  Obstacle_off_ value/1 -> Operator1/2
  Operator1/1 -> obstacle _om_off/2
  detection_obstacle/1 -> obstacle/1  "obstacle_detection"
  Unit Delay/1 -> detection_obstacle/2
  obstacle_position/1 -> Operator1/1, Operator/2
  move_up/1 -> Unit Delay/1
  window_position/1 -> Operator/1
  Operator/1 -> obstacle _om_off/1

== stateflow chart powerwindow_tl/PowerWindowController/Subsystem/PowerWindowController/control ==
  settings: description=$TL$ stepfunctionclass=STATIC_FCN; date=20160819T153442; $TL$
  state systemNormal [parallel]
    settings: executionOrder=1
    state safe
      state driverNeutral
        entry:
        moveUp = 0;
        moveDown = 0;
        state passengerneutral
          entry:
          moveUp = 0;
          moveDown = 0;
          mode = 0;
        state passengerDown
          entry: moveDown = 1;
          exit: moveDown = 0;
          state iniPassengerDown
            entry:
            mode = 2;
          state autoPassengerDown
            entry:
            mode =4;
          state passengerDown
            entry:
            mode = 2;
          iniPassengerDown -> (junction 54) : after(auto_down_time,tick)
          (junction 54) -> systemNormal.safe.driverNeutral.passengerDown.passengerDown [order 2]
          (junction 54) -> autoPassengerDown [order 1] : [passenger_neutral]
        state passengerUp
          entry: moveUp = 1;
          exit: moveUp = 0;
          state iniPassengerUp
            entry:
            mode = 1;
          state PassengerUp
            entry:
            mode = 1;
          state autoPassengerUp
            entry:
            mode =3;
          iniPassengerUp -> (junction 55) : after(auto_up_time,tick)
          (junction 55) -> PassengerUp [order 2]
          (junction 55) -> autoPassengerUp [order 1] : [passenger_neutral]
        (default) -> passengerneutral
        passengerneutral -> iniPassengerUp [order 1] : [passenger_up]
        passengerneutral -> iniPassengerDown [order 2] : [passenger_down]
        PassengerUp -> passengerneutral : [passenger_neutral]
        systemNormal.safe.driverNeutral.passengerDown.passengerDown -> passengerneutral : [passenger_neutral]
        systemNormal.safe.driverNeutral.passengerDown -> passengerneutral [order 1] : [endstop_bottom]
        passengerUp -> passengerneutral [order 2] : [endstop_top]
        systemNormal.safe.driverNeutral.passengerDown -> PassengerUp [order 2] : [passenger_up]
        passengerUp -> systemNormal.safe.driverNeutral.passengerDown.passengerDown [order 1] : [passenger_down]
      state driverDown
        entry: moveDown = 1;
        exit: moveDown = 0;
        state iniDriverDown
          entry:
          mode = 2;
        state DriverDown
          entry:
          mode = 2;
        state autoDriverDown
          entry:
          mode = 4;
        iniDriverDown -> (junction 56) : after(auto_down_time,tick)
        (junction 56) -> DriverDown [order 2]
        (junction 56) -> autoDriverDown [order 1] : [driver_neutral]
      state driverUp
        entry: moveUp = 1;
        exit: moveUp = 0;
        state iniDriverUp
          entry:
          mode = 1;
        state DriverUp
          entry:
          mode =1;
        state autoDriverUp
          entry:
          mode = 3;
        iniDriverUp -> (junction 57) : after(auto_up_time,tick)
        (junction 57) -> autoDriverUp [order 1] : [driver_neutral]
        (junction 57) -> DriverUp [order 2]
      (default) -> driverNeutral
      driverNeutral -> iniDriverDown [order 3] : [driver_down]
      DriverDown -> driverNeutral : [driver_neutral]
      driverDown -> driverNeutral [order 1] : [endstop_bottom]
      DriverUp -> driverNeutral : [driver_neutral]
      driverUp -> driverNeutral [order 2] : [endstop_top]
      driverNeutral -> iniDriverUp [order 2] : [driver_up]
      driverDown -> DriverUp [order 2] : [driver_up]
      driverUp -> DriverDown [order 1] : [driver_down]
    state emergencyDown
      entry:
      moveUp = 0;
      moveDown = 1;
      mode = 5;
    state systemError
      entry:
      mode = 100;
      moveUp = 0;
      moveDown = 0;
    emergencyDown -> passengerneutral [order 2] : [endstop_bottom | after(emergency_down_time,tick)]
    (default) -> safe
    emergencyDown -> systemError [order 1] : [counter >= 100]
    driverNeutral -> emergencyDown [order 1] : [obstacle]
    safe -> systemError : [counter >= 100]
  state obstacleDetectionCounter [parallel]
    settings: executionOrder=2
    obstacleDetectionCounter -> obstacleDetectionCounter [order 2] : [obstacle]/counter = counter +1;
    obstacleDetectionCounter -> obstacleDetectionCounter [order 1] : [!obstacle]/counter = 0;
  (default) -> systemNormal [order 1]
  (default) -> obstacleDetectionCounter [order 2]
  data: auto_up_time input; auto_down_time input; emergency_down_time input; driver_neutral input boolean; driver_up input boolean; driver_down input boolean; passenger_neutral input boolean; passenger_up input boolean; passenger_down input boolean; moveDown output boolean; moveUp output boolean; obstacle input boolean; endstop_bottom input boolean; endstop_top input boolean; mode output uint8; counter local uint8
  data auto_up_time settings: description=$TL$ type=UInt8; $TL$
  data auto_down_time settings: description=$TL$ type=UInt8; $TL$
  data emergency_down_time settings: description=$TL$ type=UInt8; $TL$
  data driver_neutral settings: description=$TL$ type=Bool; $TL$
  data driver_up settings: description=$TL$ type=Bool; $TL$
  data driver_down settings: description=$TL$ type=Bool; $TL$
  data passenger_neutral settings: description=$TL$ type=Bool; $TL$
  data passenger_up settings: description=$TL$ type=Bool; $TL$
  data passenger_down settings: description=$TL$ type=Bool; $TL$
  data moveDown settings: description=$TL$ type=Bool; $TL$
  data moveUp settings: description=$TL$ type=Bool; $TL$
  data obstacle settings: description=$TL$ type=Bool; $TL$
  data endstop_bottom settings: description=$TL$ type=Bool; $TL$
  data endstop_top settings: description=$TL$ type=Bool; $TL$
  data mode settings: description=$TL$ type=UInt8; $TL$
  data counter settings: description=$TL$ type=UInt8; $TL$
